simulink model "UAV_DONE"  (R2018a)
settings: Solver=VariableStepAuto  StartTime=0.0  StopTime=8  RelTol=1e-4
libraries: simulink x7
settings Model: Creator=Ray_X  LastModifiedBy=Ray_X

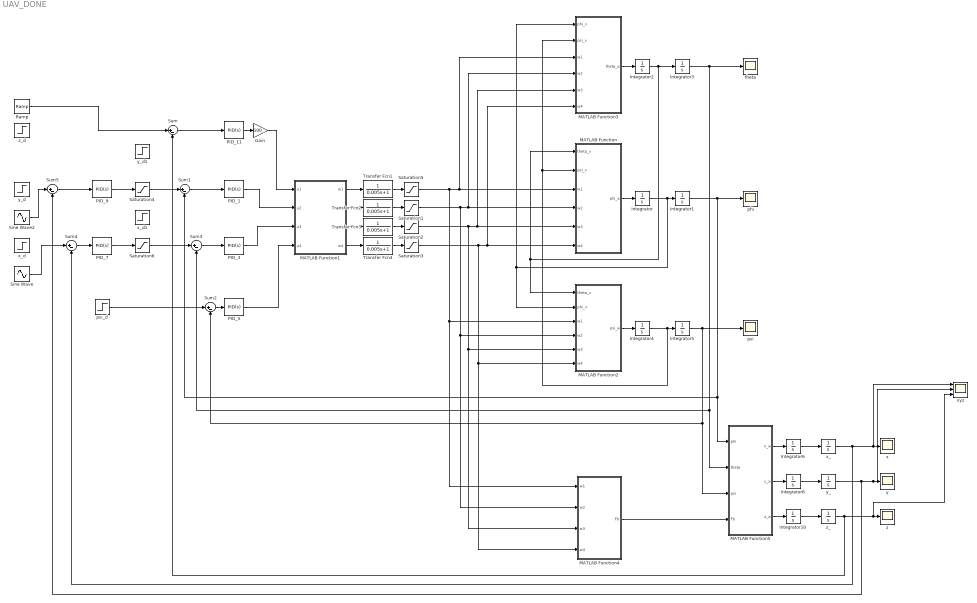
== system UAV_DONE ==
  Gain : Gain  Gain=100
  Integrator{,1..6,8,10} (9 alike) : Integrator
  MATLAB Function : MATLAB Function  TreatAsAtomicUnit=on
  MATLAB Function1 : MATLAB Function  TreatAsAtomicUnit=on
  MATLAB Function2 : MATLAB Function  TreatAsAtomicUnit=on
  MATLAB Function3 : MATLAB Function  TreatAsAtomicUnit=on
  MATLAB Function4 : MATLAB Function  TreatAsAtomicUnit=on
  MATLAB Function5 : MATLAB Function  TreatAsAtomicUnit=on
  PID_1 : simulink/Continuous/PID Controller  Controller=PID  TimeDomain=Continuous-time  SampleTime=-1  IntegratorMethod=Forward Euler  FilterMethod=Forward Euler  Form=Parallel  UseFilter=on  ControllerParametersSource=internal  P=0.17172  I=0.1  D=0.03876  N=10000  InitialConditionSource=internal  InitialConditionForIntegrator=0  InitialConditionForFilter=0  ExternalReset=none  LimitOutput=off  UpperSaturationLimit=inf  LowerSaturationLimit=-inf  LinearizeAsGain=on  AntiWindupMode=none  Kb=1  TrackingMode=off  Kt=1  PParamMin=[]  PParamMax=[]  IParamMin=[]  IParamMax=[]  DParamMin=[]  DParamMax=[]  NParamMin=[]  NParamMax=[]  KbParamMin=[]  KbParamMax=[]  KtParamMin=[]  KtParamMax=[]  POutMin=[]  POutMax=[]  IOutMin=[]  IOutMax=[]  DOutMin=[]  DOutMax=[]  NOutMin=[]  NOutMax=[]  KbOutMin=[]  KbOutMax=[]  KtOutMin=[]  KtOutMax=[]  IntegratorOutMin=[]  IntegratorOutMax=[]  FilterOutMin=[]  FilterOutMax=[]  SumOutMin=[]  SumOutMax=[]  SumI1OutMin=[]  SumI1OutMax=[]  SumI2OutMin=[]  SumI2OutMax=[]  SumI3OutMin=[]  SumI3OutMax=[]  SumDOutMin=[]  SumDOutMax=[]  SaturationOutMin=[]  SaturationOutMax=[]  IntegratorContinuousStateAttributes=''  IntegratorStateMustResolveToSignalObject=off  IntegratorRTWStateStorageClass=Auto  FilterContinuousStateAttributes=''  FilterStateMustResolveToSignalObject=off  FilterRTWStateStorageClass=Auto  DifferentiatorICPrevScaledInput=0  DifferentiatorOutMin=[]  DifferentiatorOutMax=[]  FilterDiffOutCoefMin=[]  FilterDiffOutCoefMax=[]  SumDenOutMin=[]  SumDenOutMax=[]  SumNumOutMin=[]  SumNumOutMax=[]  ReciprocalOutMin=[]  ReciprocalOutMax=[]  DivideOutMin=[]  DivideOutMax=[]  TunerSelectOption=Transfer Function Based (PID Tuner App)
  PID_11 : simulink/Continuous/PID Controller  Controller=PID  TimeDomain=Continuous-time  SampleTime=-1  IntegratorMethod=Forward Euler  FilterMethod=Forward Euler  Form=Parallel  UseFilter=on  ControllerParametersSource=internal  P=0.9944  I=1  D=0.1880  N=10000  InitialConditionSource=internal  InitialConditionForIntegrator=0  InitialConditionForFilter=0  ExternalReset=none  LimitOutput=off  UpperSaturationLimit=inf  LowerSaturationLimit=-inf  LinearizeAsGain=on  AntiWindupMode=none  Kb=1  TrackingMode=off  Kt=1  PParamMin=[]  PParamMax=[]  IParamMin=[]  IParamMax=[]  DParamMin=[]  DParamMax=[]  NParamMin=[]  NParamMax=[]  KbParamMin=[]  KbParamMax=[]  KtParamMin=[]  KtParamMax=[]  POutMin=[]  POutMax=[]  IOutMin=[]  IOutMax=[]  DOutMin=[]  DOutMax=[]  NOutMin=[]  NOutMax=[]  KbOutMin=[]  KbOutMax=[]  KtOutMin=[]  KtOutMax=[]  IntegratorOutMin=[]  IntegratorOutMax=[]  FilterOutMin=[]  FilterOutMax=[]  SumOutMin=[]  SumOutMax=[]  SumI1OutMin=[]  SumI1OutMax=[]  SumI2OutMin=[]  SumI2OutMax=[]  SumI3OutMin=[]  SumI3OutMax=[]  SumDOutMin=[]  SumDOutMax=[]  SaturationOutMin=[]  SaturationOutMax=[]  IntegratorContinuousStateAttributes=''  IntegratorStateMustResolveToSignalObject=off  IntegratorRTWStateStorageClass=Auto  FilterContinuousStateAttributes=''  FilterStateMustResolveToSignalObject=off  FilterRTWStateStorageClass=Auto  DifferentiatorICPrevScaledInput=0  DifferentiatorOutMin=[]  DifferentiatorOutMax=[]  FilterDiffOutCoefMin=[]  FilterDiffOutCoefMax=[]  SumDenOutMin=[]  SumDenOutMax=[]  SumNumOutMin=[]  SumNumOutMax=[]  ReciprocalOutMin=[]  ReciprocalOutMax=[]  DivideOutMin=[]  DivideOutMax=[]  TunerSelectOption=Transfer Function Based (PID Tuner App)
  PID_3 : simulink/Continuous/PID Controller  Controller=PID  TimeDomain=Continuous-time  SampleTime=-1  IntegratorMethod=Forward Euler  FilterMethod=Forward Euler  Form=Parallel  UseFilter=on  ControllerParametersSource=internal  P=0.18833  I=0.1  D=0.04321  N=10000  InitialConditionSource=internal  InitialConditionForIntegrator=0  InitialConditionForFilter=0  ExternalReset=none  LimitOutput=off  UpperSaturationLimit=inf  LowerSaturationLimit=-inf  LinearizeAsGain=on  AntiWindupMode=none  Kb=1  TrackingMode=off  Kt=1  PParamMin=[]  PParamMax=[]  IParamMin=[]  IParamMax=[]  DParamMin=[]  DParamMax=[]  NParamMin=[]  NParamMax=[]  KbParamMin=[]  KbParamMax=[]  KtParamMin=[]  KtParamMax=[]  POutMin=[]  POutMax=[]  IOutMin=[]  IOutMax=[]  DOutMin=[]  DOutMax=[]  NOutMin=[]  NOutMax=[]  KbOutMin=[]  KbOutMax=[]  KtOutMin=[]  KtOutMax=[]  IntegratorOutMin=[]  IntegratorOutMax=[]  FilterOutMin=[]  FilterOutMax=[]  SumOutMin=[]  SumOutMax=[]  SumI1OutMin=[]  SumI1OutMax=[]  SumI2OutMin=[]  SumI2OutMax=[]  SumI3OutMin=[]  SumI3OutMax=[]  SumDOutMin=[]  SumDOutMax=[]  SaturationOutMin=[]  SaturationOutMax=[]  IntegratorContinuousStateAttributes=''  IntegratorStateMustResolveToSignalObject=off  IntegratorRTWStateStorageClass=Auto  FilterContinuousStateAttributes=''  FilterStateMustResolveToSignalObject=off  FilterRTWStateStorageClass=Auto  DifferentiatorICPrevScaledInput=0  DifferentiatorOutMin=[]  DifferentiatorOutMax=[]  FilterDiffOutCoefMin=[]  FilterDiffOutCoefMax=[]  SumDenOutMin=[]  SumDenOutMax=[]  SumNumOutMin=[]  SumNumOutMax=[]  ReciprocalOutMin=[]  ReciprocalOutMax=[]  DivideOutMin=[]  DivideOutMax=[]  TunerSelectOption=Transfer Function Based (PID Tuner App)
  PID_5 : simulink/Continuous/PID Controller  Controller=PID  TimeDomain=Continuous-time  SampleTime=-1  IntegratorMethod=Forward Euler  FilterMethod=Forward Euler  Form=Parallel  UseFilter=on  ControllerParametersSource=internal  P=4.0510  I=1  D=0.7891  N=10000  InitialConditionSource=internal  InitialConditionForIntegrator=0  InitialConditionForFilter=0  ExternalReset=none  LimitOutput=off  UpperSaturationLimit=inf  LowerSaturationLimit=-inf  LinearizeAsGain=on  AntiWindupMode=none  Kb=1  TrackingMode=off  Kt=1  PParamMin=[]  PParamMax=[]  IParamMin=[]  IParamMax=[]  DParamMin=[]  DParamMax=[]  NParamMin=[]  NParamMax=[]  KbParamMin=[]  KbParamMax=[]  KtParamMin=[]  KtParamMax=[]  POutMin=[]  POutMax=[]  IOutMin=[]  IOutMax=[]  DOutMin=[]  DOutMax=[]  NOutMin=[]  NOutMax=[]  KbOutMin=[]  KbOutMax=[]  KtOutMin=[]  KtOutMax=[]  IntegratorOutMin=[]  IntegratorOutMax=[]  FilterOutMin=[]  FilterOutMax=[]  SumOutMin=[]  SumOutMax=[]  SumI1OutMin=[]  SumI1OutMax=[]  SumI2OutMin=[]  SumI2OutMax=[]  SumI3OutMin=[]  SumI3OutMax=[]  SumDOutMin=[]  SumDOutMax=[]  SaturationOutMin=[]  SaturationOutMax=[]  IntegratorContinuousStateAttributes=''  IntegratorStateMustResolveToSignalObject=off  IntegratorRTWStateStorageClass=Auto  FilterContinuousStateAttributes=''  FilterStateMustResolveToSignalObject=off  FilterRTWStateStorageClass=Auto  DifferentiatorICPrevScaledInput=0  DifferentiatorOutMin=[]  DifferentiatorOutMax=[]  FilterDiffOutCoefMin=[]  FilterDiffOutCoefMax=[]  SumDenOutMin=[]  SumDenOutMax=[]  SumNumOutMin=[]  SumNumOutMax=[]  ReciprocalOutMin=[]  ReciprocalOutMax=[]  DivideOutMin=[]  DivideOutMax=[]  TunerSelectOption=Transfer Function Based (PID Tuner App)
  PID_7 : simulink/Continuous/PID Controller  Controller=PID  TimeDomain=Continuous-time  SampleTime=-1  IntegratorMethod=Forward Euler  FilterMethod=Forward Euler  Form=Parallel  UseFilter=on  ControllerParametersSource=internal  P=1.65  I=0  D=0.47  N=100  InitialConditionSource=internal  InitialConditionForIntegrator=0  InitialConditionForFilter=0  ExternalReset=none  LimitOutput=off  UpperSaturationLimit=inf  LowerSaturationLimit=-inf  LinearizeAsGain=on  AntiWindupMode=none  Kb=1  TrackingMode=off  Kt=1  PParamMin=[]  PParamMax=[]  IParamMin=[]  IParamMax=[]  DParamMin=[]  DParamMax=[]  NParamMin=[]  NParamMax=[]  KbParamMin=[]  KbParamMax=[]  KtParamMin=[]  KtParamMax=[]  POutMin=[]  POutMax=[]  IOutMin=[]  IOutMax=[]  DOutMin=[]  DOutMax=[]  NOutMin=[]  NOutMax=[]  KbOutMin=[]  KbOutMax=[]  KtOutMin=[]  KtOutMax=[]  IntegratorOutMin=[]  IntegratorOutMax=[]  FilterOutMin=[]  FilterOutMax=[]  SumOutMin=[]  SumOutMax=[]  SumI1OutMin=[]  SumI1OutMax=[]  SumI2OutMin=[]  SumI2OutMax=[]  SumI3OutMin=[]  SumI3OutMax=[]  SumDOutMin=[]  SumDOutMax=[]  SaturationOutMin=[]  SaturationOutMax=[]  IntegratorContinuousStateAttributes=''  IntegratorStateMustResolveToSignalObject=off  IntegratorRTWStateStorageClass=Auto  FilterContinuousStateAttributes=''  FilterStateMustResolveToSignalObject=off  FilterRTWStateStorageClass=Auto  DifferentiatorICPrevScaledInput=0  DifferentiatorOutMin=[]  DifferentiatorOutMax=[]  FilterDiffOutCoefMin=[]  FilterDiffOutCoefMax=[]  SumDenOutMin=[]  SumDenOutMax=[]  SumNumOutMin=[]  SumNumOutMax=[]  ReciprocalOutMin=[]  ReciprocalOutMax=[]  DivideOutMin=[]  DivideOutMax=[]  TunerSelectOption=Transfer Function Based (PID Tuner App)
  PID_9 : simulink/Continuous/PID Controller  Controller=PID  TimeDomain=Continuous-time  SampleTime=-1  IntegratorMethod=Forward Euler  FilterMethod=Forward Euler  Form=Parallel  UseFilter=on  ControllerParametersSource=internal  P=1.65  I=0  D=0.47  N=100  InitialConditionSource=internal  InitialConditionForIntegrator=0  InitialConditionForFilter=0  ExternalReset=none  LimitOutput=off  UpperSaturationLimit=inf  LowerSaturationLimit=-inf  LinearizeAsGain=on  AntiWindupMode=none  Kb=1  TrackingMode=off  Kt=1  PParamMin=[]  PParamMax=[]  IParamMin=[]  IParamMax=[]  DParamMin=[]  DParamMax=[]  NParamMin=[]  NParamMax=[]  KbParamMin=[]  KbParamMax=[]  KtParamMin=[]  KtParamMax=[]  POutMin=[]  POutMax=[]  IOutMin=[]  IOutMax=[]  DOutMin=[]  DOutMax=[]  NOutMin=[]  NOutMax=[]  KbOutMin=[]  KbOutMax=[]  KtOutMin=[]  KtOutMax=[]  IntegratorOutMin=[]  IntegratorOutMax=[]  FilterOutMin=[]  FilterOutMax=[]  SumOutMin=[]  SumOutMax=[]  SumI1OutMin=[]  SumI1OutMax=[]  SumI2OutMin=[]  SumI2OutMax=[]  SumI3OutMin=[]  SumI3OutMax=[]  SumDOutMin=[]  SumDOutMax=[]  SaturationOutMin=[]  SaturationOutMax=[]  IntegratorContinuousStateAttributes=''  IntegratorStateMustResolveToSignalObject=off  IntegratorRTWStateStorageClass=Auto  FilterContinuousStateAttributes=''  FilterStateMustResolveToSignalObject=off  FilterRTWStateStorageClass=Auto  DifferentiatorICPrevScaledInput=0  DifferentiatorOutMin=[]  DifferentiatorOutMax=[]  FilterDiffOutCoefMin=[]  FilterDiffOutCoefMax=[]  SumDenOutMin=[]  SumDenOutMax=[]  SumNumOutMin=[]  SumNumOutMax=[]  ReciprocalOutMin=[]  ReciprocalOutMax=[]  DivideOutMin=[]  DivideOutMax=[]  TunerSelectOption=Transfer Function Based (PID Tuner App)
  Ramp : simulink/Sources/Ramp  slope=0.5  start=0  InitialOutput=0
  Saturation{1..3,5} (4 alike) : Saturate  UpperLimit=2600*2600  LowerLimit=-2600*2600
  Saturation4 : Saturate  UpperLimit=1.5  LowerLimit=-1.5
  Saturation6 : Saturate  UpperLimit=1.5  LowerLimit=-1.5
  Sine Wave : Sin  Frequency=1*pi()  SampleTime=0
  Sine Wave2 : Sin  Frequency=1*pi()  Phase=pi()/2  SampleTime=0
  Sum{,1..5} (6 alike) : Sum  Inputs=|+-
  Transfer Fcn{1..4} (4 alike) : TransferFcn  Denominator=[0.005 1]
  phi : Scope
  psi : Scope
  psi_d : Step  After=0  SampleTime=0
  theta : Scope
  x : Scope
  x_ : Integrator
  x_d : Step  Time=3  SampleTime=0
  x_d1 : Step  SampleTime=0
  xyz : Scope  NumInputPorts=3
  y : Scope
  y_ : Integrator
  y_d : Step  Time=3  SampleTime=0
  y_d1 : Step  SampleTime=0
  z : Scope
  z_ : Integrator
  z_d : Step  Time=5  After=0  SampleTime=0
  wires:
  MATLAB Function/1(phi_a) -> Integrator/1
  Integrator/1 -> MATLAB Function2/2(phi_v), MATLAB Function3/1(phi_v), Integrator1/1
  MATLAB Function3/1(theta_a) -> Integrator2/1
  MATLAB Function2/1(psi_a) -> Integrator4/1
  PID_5/1 -> MATLAB Function1/4(u4)
  PID_1/1 -> MATLAB Function1/2(u2)
  PID_3/1 -> MATLAB Function1/3(u3)
  Integrator3/1 -> MATLAB Function5/2(theta), Sum3/2, theta/1
  Integrator1/1 -> MATLAB Function5/1(phi), Sum1/2, phi/1
  Integrator5/1 -> MATLAB Function5/3(psi), Sum2/2, psi/1
  MATLAB Function4/1(Fti) -> MATLAB Function5/4(Fti)
  Sum1/1 -> PID_1/1
  Sum3/1 -> PID_3/1
  Sum2/1 -> PID_5/1
  psi_d/1 -> Sum2/1
  MATLAB Function5/1(x_a) -> Integrator6/1
  Integrator6/1 -> x_/1
  x_/1 -> Sum4/2, xyz/1, x/1
  MATLAB Function5/2(y_a) -> Integrator8/1
  Integrator8/1 -> y_/1
  MATLAB Function5/3(z_a) -> Integrator10/1
  z_/1 -> xyz/3, z/1, Sum/2
  Integrator10/1 -> z_/1
  Integrator2/1 -> MATLAB Function2/1(theta_v), MATLAB Function/1(theta_v), Integrator3/1
  Integrator4/1 -> Integrator5/1, MATLAB Function3/2(psi_v), MATLAB Function/2(psi_v)
  MATLAB Function1/1(w1) -> Transfer Fcn1/1
  MATLAB Function1/4(w4) -> Transfer Fcn4/1
  MATLAB Function1/3(w3) -> Transfer Fcn3/1
  MATLAB Function1/2(w2) -> Transfer Fcn2/1
  Transfer Fcn1/1 -> Saturation5/1
  Saturation5/1 -> MATLAB Function4/1(w1), MATLAB Function2/3(w1), MATLAB Function/3(w1), MATLAB Function3/3(w1)
  Saturation3/1 -> MATLAB Function3/6(w4), MATLAB Function/6(w4), MATLAB Function2/6(w4), MATLAB Function4/4(w4)
  Saturation2/1 -> MATLAB Function3/5(w3), MATLAB Function/5(w3), MATLAB Function2/5(w3), MATLAB Function4/3(w3)
  Saturation1/1 -> MATLAB Function/4(w2), MATLAB Function3/4(w2), MATLAB Function4/2(w2), MATLAB Function2/4(w2)
  Transfer Fcn4/1 -> Saturation3/1
  Transfer Fcn3/1 -> Saturation2/1
  Transfer Fcn2/1 -> Saturation1/1
  Gain/1 -> MATLAB Function1/1(u1)
  Sum4/1 -> PID_7/1
  Sum5/1 -> PID_9/1
  PID_7/1 -> Saturation6/1
  PID_9/1 -> Saturation4/1
  y_/1 -> Sum5/2, xyz/2, y/1
  Sum/1 -> PID_11/1
  PID_11/1 -> Gain/1
  Saturation4/1 -> Sum1/1
  Saturation6/1 -> Sum3/1
  Ramp/1 -> Sum/1
  Sine Wave/1 -> Sum4/1
  Sine Wave2/1 -> Sum5/1

== matlab function UAV_DONE/MATLAB Function1 ==
  data: u1 input; w1 output; u2 input; u3 input; u4 input; w2 output; w3 output; w4 output
function [w1,w2,w3,w4] = U2w(u1,u2,u3,u4)
b=3.13*1e-5;
d=7.5*1e-7;
l=0.2;
bl=b*l;
Bd=[b b b b
    0 -bl 0 bl
    -bl 0 bl 0
    -d d -d d];
U=[u1,u2,u3,u4]';
w=Bd^-1*U;
w1=w(1);
w2=w(2);
w3=w(3);
w4=w(4);

== matlab function UAV_DONE/MATLAB Function ==
  data: theta_v input; psi_v input; w1 input; phi_a output; w2 input; w3 input; w4 input
function phi_a = phi_a(theta_v,psi_v,w1,w2,w3,w4)
IXX=2.353*1e-3;
IYY=2.635*1e-3;
IZZ=5.262*1e-2;
l=0.2;
b=3.13*1e-5;
JR=6*1e-5;

T=b*l*(w4-w2);

W1=real(sqrt(complex(w1)));
W2=real(sqrt(complex(w2)));
W3=real(sqrt(complex(w3)));
W4=real(sqrt(complex(w4)));
WR=-W1+W2-W3+W4;

phi_a=theta_v*psi_v*(IYY-IZZ)/IXX;
phi_a=phi_a+JR*theta_v*WR/IXX;
phi_a=phi_a+T/IXX;

== matlab function UAV_DONE/MATLAB Function2 ==
  data: theta_v input; phi_v input; w1 input; psi_a output; w2 input; w3 input; w4 input
function psi_a = psi_a(theta_v,phi_v,w1,w2,w3,w4)
IXX=2.353*1e-3;
IYY=2.635*1e-3;
IZZ=5.262*1e-2;
d=7.5*1e-7;

M1=d*w1;
M2=d*w2;
M3=d*w3;
M4=d*w4;
M=-M1+M2-M3+M4;

psi_a=theta_v*phi_v*(IXX-IYY)/IZZ;
psi_a=psi_a+M/IZZ;

== matlab function UAV_DONE/MATLAB Function3 ==
  data: phi_v input; psi_v input; w1 input; theta_a output; w2 input; w3 input; w4 input
function theta_a = theta_a(phi_v,psi_v,w1,w2,w3,w4)
IXX=2.353*1e-3;
IYY=2.635*1e-3;
IZZ=5.262*1e-2;
l=0.2;
b=3.13*1e-5;
JR=6*1e-5;

T=b*l*(w3-w1);

W1=real(sqrt(complex(w1)));
W2=real(sqrt(complex(w2)));
W3=real(sqrt(complex(w3)));
W4=real(sqrt(complex(w4)));
WR=-W1+W2-W3+W4;

theta_a=phi_v*psi_v*(IZZ-IXX)/IYY;
theta_a=theta_a-JR*phi_v*WR/IYY;
theta_a=theta_a+T/IYY;

== matlab function UAV_DONE/MATLAB Function4 ==
  data: w1 input; Fti output; w2 input; w3 input; w4 input
function Fti= Fti(w1,w2,w3,w4)
b=3.13*1e-5;
Fti=b*(w1+w2+w3+w4);

== matlab function UAV_DONE/MATLAB Function5 ==
  data: phi input; x_a output; theta input; psi input; Fti input; y_a output; z_a output
function [x_a,y_a,z_a] = xyz_a(phi,theta,psi,Fti)
m=1.2;
x_a=sin(psi)*sin(phi)+cos(psi)*sin(theta)*cos(phi);
x_a=x_a*Fti/m;

y_a=(-cos(psi)*sin(phi)+sin(psi)*sin(theta)*cos(phi));
y_a=-y_a*Fti/m;

z_a=(cos(theta)*cos(phi))*Fti/m-9.81;
